simulink model "current_source_inverter"  (Simulink 7.3)
settings: Solver=ode45  StartTime=0.0  StopTime=0.03  MaxStep=1e-3  RelTol=1e-3
InitFcn:
  | % Processor selection for I/O assignment
  | % The chosen Target in the Coder Options window must match the selected LaunchPad.
  | % Set the variable 'type_evm' to the following strings to choose a specific target:
  | 
  |   type_evm = 'TI28379LP';  % TI28379D Delfino Launchpad
  | % type_evm = 'TI28377S';   % TI28377S Delfino Launchpad
  | % type_evm = 'TI280049C';  % TI280049C Piccolo Launchpad
  | % type_evm = 'TI28379CC';  % TI28379D Delfino Controlcard
  | % type_evm = 'TI28388D';   % TI28388D Controlcard
  | 
  | % Configure I/O based on processor
  | switch (type_evm)
  | 
  | 	case 'TI28379LP'
  | 	% Configuration for TI28379D Launchpad
  | 	% On the Plant side
  | 		PWMCAP_RTBox = [0 2 4 16 18 20];
  | 		AO_Factor = 1;
  | 		AO_Vmax = 3.3;
  | 
  | 	% On the MCU side
  | 		PWM_DSP = [1:6];
  | 		DO_DSP_LED = 34;
  |       SCI_DSP = [43,42];
  | 
  | 	case 'TI28377S'
  | 	% Configuration for TI28377S Launchpad
  | 	% On the Plant side
  | 		PWMCAP_RTBox = [16 18 0 2 4 20];
  | 		AO_Factor = 1;
  | 		AO_Vmax = 3.3;
  | 
  | 	% On the MCU side
  | 		PWM_DSP = [2 6 7 8 9 10];
  | 		DO_DSP_LED = 13;
  |       SCI_DSP = [85,84];
  | 
  | 	case 'TI280049C'
  | 	% Configuration for TI280049C Launchpad
  | 	% On the Plant side
  | 		PWMCAP_RTBox = [0 2 4 16 18 20];
  | 		AO_Factor = 1;
  | 		AO_Vmax = 3.3;
  | 
  | 	% On the MCU side
  | 		PWM_DSP = [6 5 3 1 4 2];
  | 		DO_DSP_LED = 34;
  |       SCI_DSP = [28, 29];
  | 
  | 	case 'TI28379CC'
  | 	% Configuration for TI28379D Controlcard
  | 	% On the Plant side
  | 		PWMCAP_RTBox =  [0,2,4,6,8,10];
  | 		AO_Factor = 1.54; % breakout board scaling 6.8k/4.42k
  | 		AO_Vmax = 5.0;
  | 
  | 	% On the MCU side
  | 		PWM_DSP = 1:6;
  | 		DO_DSP_LED = 34;
  | 		SCI_DSP = [28, 29];
  | 
  | 
  | 		case 'TI28388D'
  | 	% Configuration for TI28388D Controlcard
  | 	% On the Plant side
  | 		PWMCAP_RTBox = [0,2,4,6,8,10];
  | 		AO_Factor = 1.54; % breakout board scaling 6.8k/4.42k
  | 		AO_Vmax = 5.0;
  | 
  | 	% On the MCU side
  | 		PWM_DSP = 1:6;
  | 		DO_DSP_LED = 34;
  | 		SCI_DSP = [28, 29];
  | 
  | 	otherwise
  | 	error('Unknown evaluation module selection, please choose either ''TI28377S'', ''TI28379LP'', ''TI280049C'', ''TI28379CC'' or ''TI28388D''.')
  | end
  | 
  | fsw = 20e3;
  | fgrid = 50;
  | Tdisc.plant = 3e-6;
  | Tdisc.ctrl = 1/fsw;
  | 
  | Vin = 400;
  | Po = 1e4;
  | Iin = Po/Vin;
  | Iload_pk = 20;
  | Dd = Iload_pk/Iin;
  | Iload_rms = Iload_pk/sqrt(2);
  | Rload = Po/3/(Iload_rms^2);
  | Lin = 2e-3;
  | Cf = 4.8e-6;
  | Lload = 252e-6;
undefined symbols (not defined in the file): plecs
settings Model: Creator=kris  LastModifiedBy=manaswini  ExtModeTrigMode=oneshot  ExtModeArmWhenConnect=off  ExtModeAutoUpdateStatusClock=off
settings DataIOCC: LimitDataPoints=off  ReturnWorkspaceOutputs=off  SignalLoggingName=sigsOut
settings OptimizationCC: BooleanDataType=off  ExpressionDepthLimit=128  InitFltsAndDblsToZero=on
settings DebuggingCC: SaveWithParameterizedLinksMsg=none  SignalResolutionControl=TryResolveAllWithWarning  SolverPrmCheckMsg=none  MultiTaskDSMMsg=warning  MultiTaskCondExecSysMsg=none  FcnCallInpInsideContextMsg=Enable All  StrictBusMsg=ErrorLevel1
settings HardwareCC: TargetHWDeviceType=32-bit Generic  TargetUnknown=on  ProdEqTarget=off
settings RTWCC: IncludeERTFirstTime=on
settings CodeAppCC: CustomSymbolStrType=$N$R$M_T
settings GRTTargetCC: TargetFcnLib=ansi_tfl_tmw.mat  TargetFunctionLibrary=C89/C90 (ANSI)  ModelReferenceCompliant=off

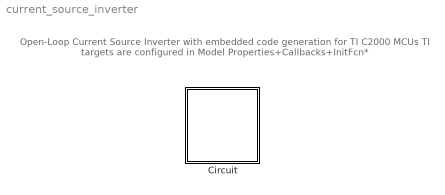
== system current_source_inverter ==
  note: Open-Loop Current Source Inverter
      | with embedded code generation for TI C2000 MCUs
      | TI targets are configured in Model Properties+Callbacks+InitFcn*
  Circuit : Subsystem  LoadFcn=plecs('sl', 200);  InitFcn=plecs('sl', 214);  StartFcn=plecs('sl', 208);  StopFcn=plecs('sl', 209);  ClipboardFcn=plecs('sl', 212, 8);  mask(PlecsCircuit){PLECSData=<binary blob, 27096 chars, not shown>}
      mask prompts: PLECSData "PLECS Data (Do not delete or modify!)"
      mask help: Drag this block into a Simulink model to create a new electrical circuit.
      mask init:
      | % PLACE CUSTOM INITIALIZATIONS ABOVE
      | % DO NOT REMOVE
      | plecs('sl', 215);
      | % DO NOT REMOVE
      settings: CopyFcn=plecs('sl', 203);  DeleteFcn=plecs('sl', 205);  UndoDeleteFcn=plecs('sl', 206);  PreSaveFcn=plecs('sl', 211);  PostSaveFcn=plecs('sl', 201);  NameChangeFcn=plecs('sl', 210);  DestroyFcn=plecs('sl', 207);  PreCopyFcn=plecs('sl', 216);  OpenFcn=plecs('sl', 202);  ErrorFcn=plerrorfcn
      mask Display: disp('PLECS\nCircuit')

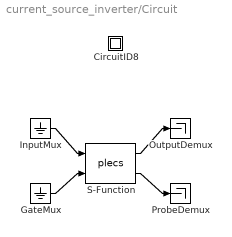
== system current_source_inverter/Circuit ==
  " CircuitID8 " : Subsystem
  " GateMux " : Ground
  " InputMux " : Ground
  " OutputDemux " : Terminator
  " ProbeDemux " : Terminator
  " S-Function " : S-Function  FunctionName=plecs  EnableBusSupport=off
  wires:
  " InputMux "/1 -> " S-Function "/1
  " GateMux "/1 -> " S-Function "/2
  " S-Function "/1 -> " OutputDemux "/1
  " S-Function "/2 -> " ProbeDemux "/1

== system current_source_inverter/Circuit/ CircuitID8  ==
